simulink model "LQR_Sim"  (R2023a)
settings: Solver=VariableStepAuto  StartTime=0.0  StopTime=10.0  RelTol=1e-3
InitFcn:
  | % 定义倒立摆相关物理量
  | L = 1;  % 倒立摆摆长
  | g = 10; % 重力加速度
  | 
  | % 定义状态空间方程相关矩阵
  | A = [0, 1; g/L, 0];
  | B = [0; -1];
  | C = [0, 1]; % 输出x2即角速度
  | D = [0];
  | 
  | % 定义QR矩阵参数
  | Q1 = diag([100, 1]); % 第一组 要求：快收敛
  | R1 = 0.01;
  | Q2 = diag([1, 1]); % 第二组 要求：小输入完成
  | R2 = 100;
  | 
  | % 计算K矩阵
  | K1 = calc_LQR_K(A, B, Q1, R1); % 第一组
  | K2 = calc_LQR_K(A, B, Q2, R2); % 第二组
model workspace (MAT data in the model file):
  initial_pos = 5
settings Model: Creator=asus  LastModifiedBy=asus

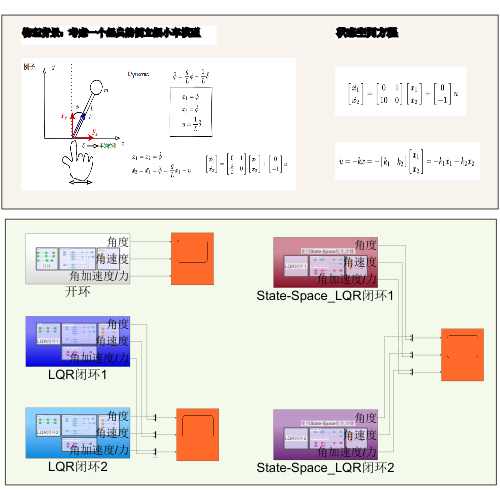
[thumbnail: Simulink's stored preview of the top-level diagram]
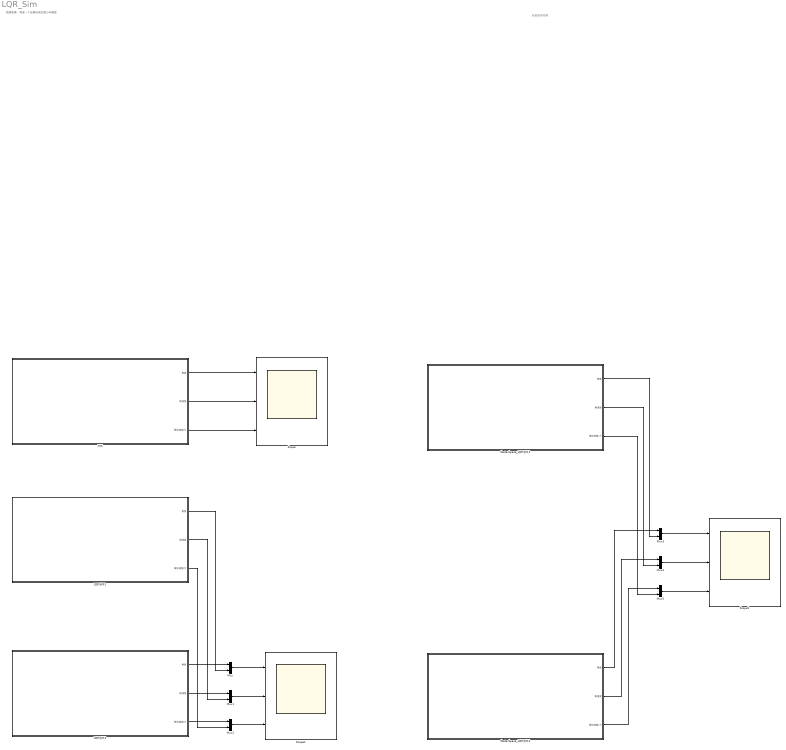
== system LQR_Sim ==
  note: 状态空间方程
  note: 物理背景：考虑一个经典的倒立摆小车模型
  LQR闭环1 : Subsystem
  LQR闭环2 : Subsystem
  Mux{,1..5} (6 alike) : Mux  Inputs=2
  Scope : Scope  NumInputPorts=3
  Scope1 : Scope  NumInputPorts=3
  Scope2 : Scope  NumInputPorts=3
  State-Space_LQR闭环1 : Subsystem
  State-Space_LQR闭环2 : Subsystem
  开环 : Subsystem
  wires:
  开环/3(角加速度/力) -> Scope/3
  开环/2(角速度) -> Scope/2
  开环/1(角度) -> Scope/1
  Mux/1 -> Scope1/1
  Mux1/1 -> Scope1/2
  Mux2/1 -> Scope1/3
  LQR闭环2/3(角加速度/力) -> Mux2/1
  LQR闭环2/2(角速度) -> Mux1/1
  LQR闭环2/1(角度) -> Mux/1
  LQR闭环1/1(角度) -> Mux/2
  LQR闭环1/2(角速度) -> Mux1/2
  LQR闭环1/3(角加速度/力) -> Mux2/2
  State-Space_LQR闭环2/3(角加速度/力) -> Mux5/1
  State-Space_LQR闭环2/1(角度) -> Mux3/1
  Mux5/1 -> Scope2/3
  Mux3/1 -> Scope2/1
  State-Space_LQR闭环1/3(角加速度/力) -> Mux5/2
  State-Space_LQR闭环1/2(角速度) -> Mux4/2
  State-Space_LQR闭环2/2(角速度) -> Mux4/1
  State-Space_LQR闭环1/1(角度) -> Mux3/2
  Mux4/1 -> Scope2/2

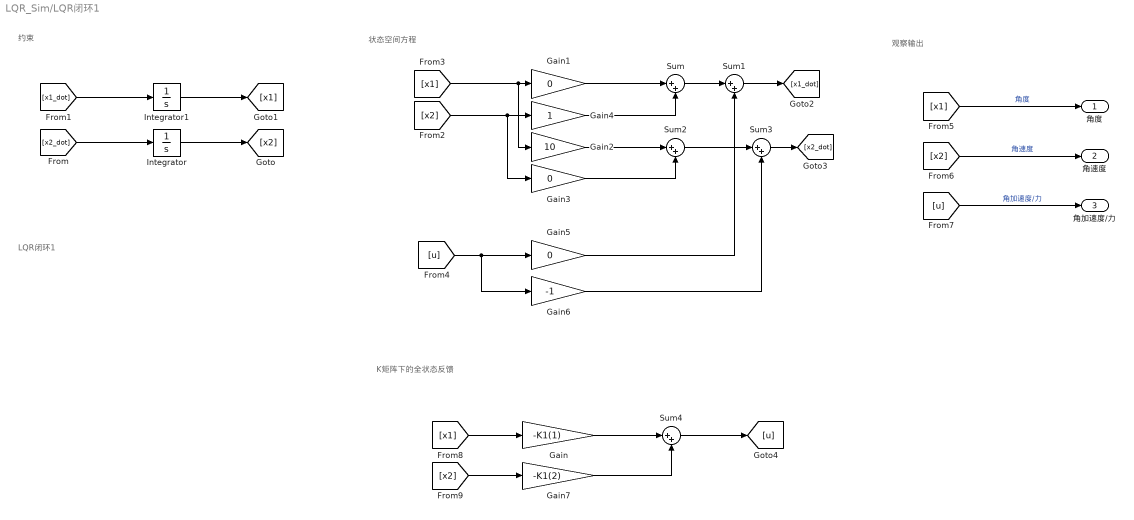
== system LQR_Sim/LQR闭环1 ==
  note: K矩阵下的全状态反馈
  note: 约束
  note: 状态空间方程
  note: 观察输出
  note: LQR闭环1
  Gain : Gain  Gain=-K1(1)
  Gain1 : Gain  Gain=0
  Gain2 : Gain  Gain=10
  Gain3 : Gain  Gain=0
  Gain4 : Gain
  Gain5 : Gain  Gain=0
  Gain6 : Gain  Gain=-1
  Gain7 : Gain  Gain=-K1(2)
  Integrator : Integrator
  Integrator1 : Integrator  InitialCondition=initial_pos
  Sum{,1..4} (5 alike) : Sum  Inputs=|++
  角度 : Outport
  角速度 : Outport  Port=2
  角加速度/力 : Outport  Port=3
  wires:
  [u] -> 角加速度/力/1  "角加速度/力"
  [x2] -> 角速度/1  "角速度"
  [x1] -> 角度/1  "角度"
  Sum3/1 -> [x2_dot]
  Gain3/1 -> Sum2/2
  Gain1/1 -> Sum/1
  Gain2/1 -> Sum2/1
  Sum1/1 -> [x1_dot]
  Integrator/1 -> [x2]
  [x1_dot] -> Integrator1/1
  [x1] -> Gain1/1, Gain2/1
  Gain4/1 -> Sum/2
  Integrator1/1 -> [x1]
  Gain6/1 -> Sum3/2
  Sum/1 -> Sum1/1
  Sum2/1 -> Sum3/1
  [x2_dot] -> Integrator/1
  Gain5/1 -> Sum1/2
  [u] -> Gain5/1, Gain6/1
  [x2] -> Gain4/1, Gain3/1
  [x1] -> Gain/1
  Gain/1 -> Sum4/1
  [x2] -> Gain7/1
  Gain7/1 -> Sum4/2
  Sum4/1 -> [u]

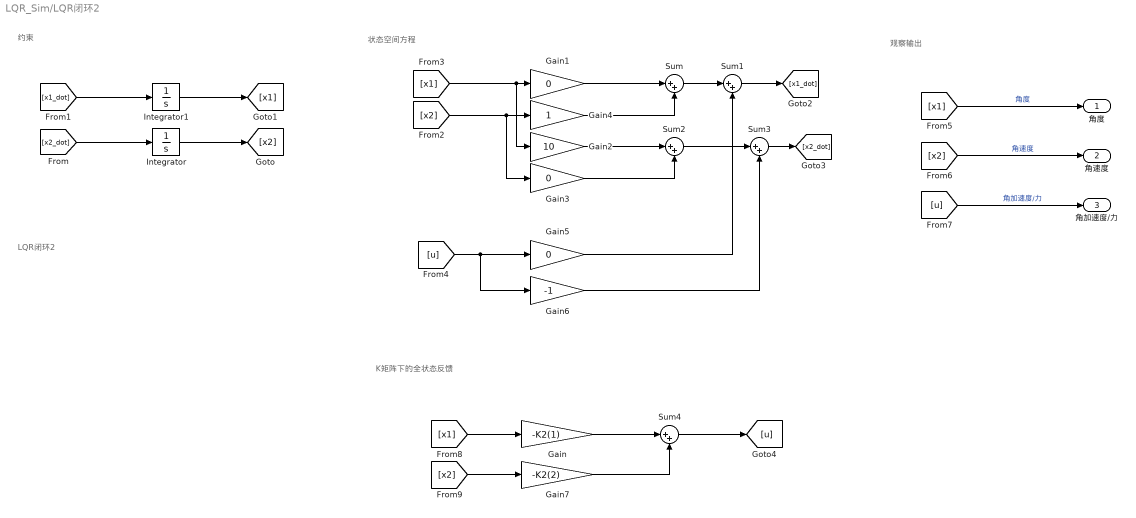
== system LQR_Sim/LQR闭环2 ==
  note: LQR闭环2
  note: 约束
  note: 状态空间方程
  note: 观察输出
  note: K矩阵下的全状态反馈
  Gain : Gain  Gain=-K2(1)
  Gain1 : Gain  Gain=0
  Gain2 : Gain  Gain=10
  Gain3 : Gain  Gain=0
  Gain4 : Gain
  Gain5 : Gain  Gain=0
  Gain6 : Gain  Gain=-1
  Gain7 : Gain  Gain=-K2(2)
  Integrator : Integrator
  Integrator1 : Integrator  InitialCondition=initial_pos
  Sum{,1..4} (5 alike) : Sum  Inputs=|++
  角度 : Outport
  角速度 : Outport  Port=2
  角加速度/力 : Outport  Port=3
  wires:
  Integrator1/1 -> [x1]
  [u] -> Gain5/1, Gain6/1
  [x1_dot] -> Integrator1/1
  Gain4/1 -> Sum/2
  Integrator/1 -> [x2]
  [x1] -> Gain1/1, Gain2/1
  Gain1/1 -> Sum/1
  Sum/1 -> Sum1/1
  [x2_dot] -> Integrator/1
  Gain6/1 -> Sum3/2
  Sum2/1 -> Sum3/1
  [x2] -> Gain4/1, Gain3/1
  [x1] -> 角度/1  "角度"
  Gain5/1 -> Sum1/2
  Gain2/1 -> Sum2/1
  Gain3/1 -> Sum2/2
  Sum1/1 -> [x1_dot]
  [x2] -> 角速度/1  "角速度"
  Gain7/1 -> Sum4/2
  [x2] -> Gain7/1
  Gain/1 -> Sum4/1
  Sum3/1 -> [x2_dot]
  [x1] -> Gain/1
  Sum4/1 -> [u]
  [u] -> 角加速度/力/1  "角加速度/力"

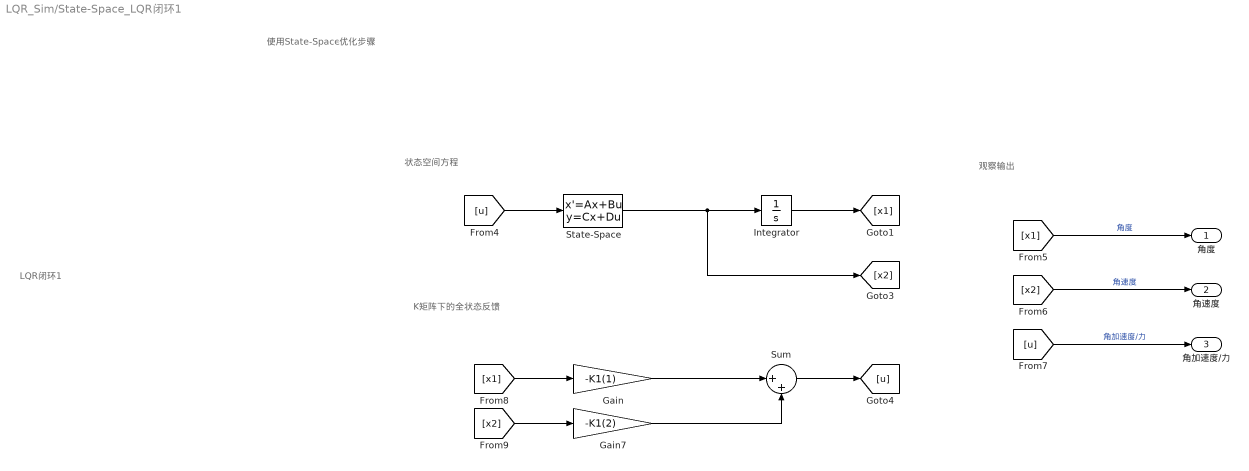
== system LQR_Sim/State-Space_LQR闭环1 ==
  note: 使用State-Space优化步骤
  note: K矩阵下的全状态反馈
  note: 观察输出
  note: 状态空间方程
  note: LQR闭环1
  Gain : Gain  Gain=-K1(1)
  Gain7 : Gain  Gain=-K1(2)
  Integrator : Integrator  InitialCondition=initial_pos
  State-Space : StateSpace  A=A  B=B  C=C  D=D  InitialCondition=0
  Sum : Sum  Inputs=|++
  角度 : Outport
  角速度 : Outport  Port=2
  角加速度/力 : Outport  Port=3
  wires:
  [x1] -> Gain/1
  Sum/1 -> [u]
  [x2] -> Gain7/1
  [x2] -> 角速度/1  "角速度"
  [u] -> 角加速度/力/1  "角加速度/力"
  [x1] -> 角度/1  "角度"
  Integrator/1 -> [x1]
  Gain/1 -> Sum/1
  Gain7/1 -> Sum/2
  [u] -> State-Space/1
  State-Space/1 -> [x2], Integrator/1

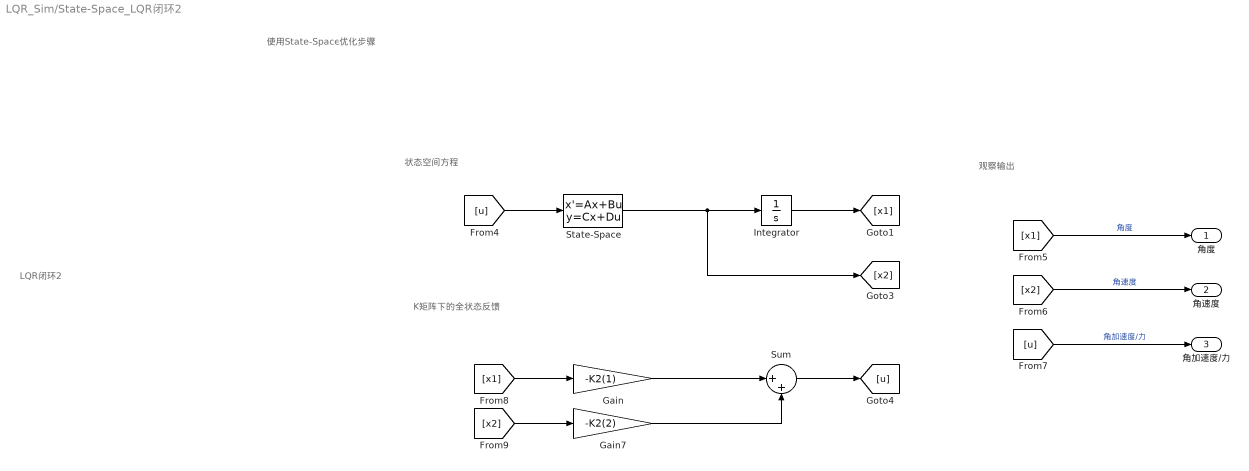
== system LQR_Sim/State-Space_LQR闭环2 ==
  note: 观察输出
  note: LQR闭环2
  note: 使用State-Space优化步骤
  note: 状态空间方程
  note: K矩阵下的全状态反馈
  Gain : Gain  Gain=-K2(1)
  Gain7 : Gain  Gain=-K2(2)
  Integrator : Integrator  InitialCondition=initial_pos
  State-Space : StateSpace  A=A  B=B  C=C  D=D  InitialCondition=0
  Sum : Sum  Inputs=|++
  角度 : Outport
  角速度 : Outport  Port=2
  角加速度/力 : Outport  Port=3
  wires:
  State-Space/1 -> [x2], Integrator/1
  Sum/1 -> [u]
  [x2] -> 角速度/1  "角速度"
  Integrator/1 -> [x1]
  [x1] -> 角度/1  "角度"
  [u] -> 角加速度/力/1  "角加速度/力"
  Gain/1 -> Sum/1
  [x2] -> Gain7/1
  [u] -> State-Space/1
  Gain7/1 -> Sum/2
  [x1] -> Gain/1

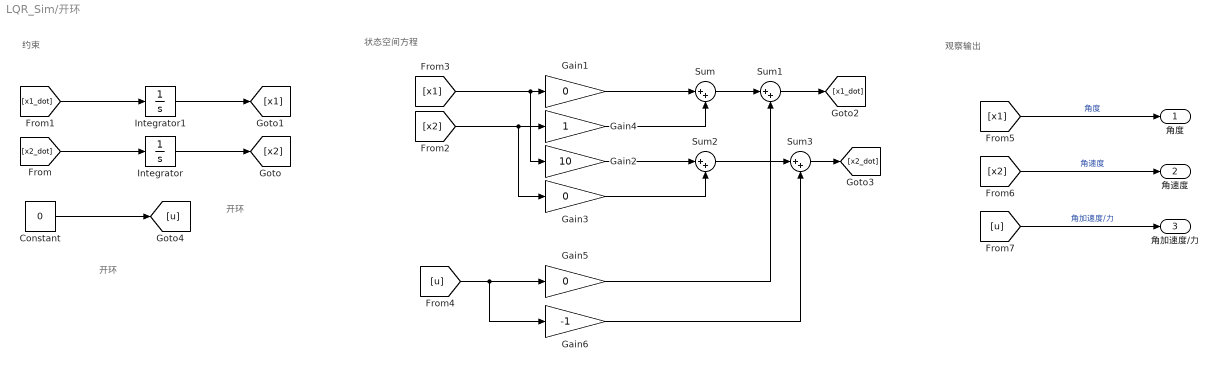
== system LQR_Sim/开环 ==
  note: 开环
  note: 观察输出
  note: 状态空间方程
  note: 开环
  note: 约束
  Constant : Constant  Value=0
  Gain1 : Gain  Gain=0
  Gain2 : Gain  Gain=10
  Gain3 : Gain  Gain=0
  Gain4 : Gain
  Gain5 : Gain  Gain=0
  Gain6 : Gain  Gain=-1
  Integrator : Integrator
  Integrator1 : Integrator  InitialCondition=initial_pos
  Sum{,1..3} (4 alike) : Sum  Inputs=|++
  角度 : Outport
  角速度 : Outport  Port=2
  角加速度/力 : Outport  Port=3
  wires:
  [x2] -> Gain3/1, Gain4/1
  [u] -> Gain6/1, Gain5/1
  Gain5/1 -> Sum1/2
  [x2_dot] -> Integrator/1
  Sum2/1 -> Sum3/1
  Sum/1 -> Sum1/1
  Gain6/1 -> Sum3/2
  Integrator1/1 -> [x1]
  Gain4/1 -> Sum/2
  [x1] -> Gain2/1, Gain1/1
  [x1_dot] -> Integrator1/1
  Integrator/1 -> [x2]
  Sum1/1 -> [x1_dot]
  Gain2/1 -> Sum2/1
  Gain1/1 -> Sum/1
  Gain3/1 -> Sum2/2
  Sum3/1 -> [x2_dot]
  Constant/1 -> [u]
  [x1] -> 角度/1  "角度"
  [x2] -> 角速度/1  "角速度"
  [u] -> 角加速度/力/1  "角加速度/力"
